simulink model "soc_pmsm_dualcpu_foc_sw_c28xCPU2"  (R2023b)
settings: Solver=FixedStepAuto  StartTime=0.0  StopTime=1  RelTol=1e-3  EnableMultiTasking=on
StartFcn:
  | warning('off', 'Simulink:Engine:ExtModeCannotDownloadParamBecauseNoHostToTarget');
StopFcn:
  | warning('on', 'Simulink:Engine:ExtModeCannotDownloadParamBecauseNoHostToTarget');
undefined symbols (not defined in the file): m, n
libraries: prociodatalib x6, proctasklib x1
settings Model: Creator=13571  LastModifiedBy=13571
settings SolverCC: AlgebraicLoopSolver=TrustRegion  PositivePriorityOrder=on  MaxZcPerStep=1
settings DataIOCC: SaveOutput=off  DSMLogging=off
settings OptimizationCC: DefaultUnderspecifiedDataType=single  EnhancedBackFolding=on  PassReuseOutputArgsAs=Individual arguments  MaxStackSize=1024  OptimizeBlockOrder=speed  DifferentSizesBufferReuse=on  OptimizationCustomize=off  DenormalBehavior=FlushToZero  EfficientTunableParamExpr=on
settings DebuggingCC: InheritedTsInSrcMsg=none  ParameterPrecisionLossMsg=none  ParameterTunabilityLossMsg=error  UnconnectedInputMsg=warning  UnconnectedOutputMsg=warning  UnconnectedLineMsg=warning
settings HardwareCC: ProdBitPerChar=16  ProdBitPerInt=16  ProdBitPerPointer=32  ProdBitPerSizeT=32  ProdBitPerPtrDiffT=32  ProdLargestAtomicInteger=Integer  ProdLargestAtomicFloat=None  ProdWordSize=16  ProdLongLongMode=on  ProdHWDeviceType=Texas Instruments->C2000  HardwareBoardFeatureSet=SoCBlockset
settings ModelReferenceCC: EnableRefExpFcnMdlSchedulingChecks=on  ModelReferenceNumInstancesAllowed=Single
settings SFSimCC: MATLABDynamicMemAlloc=off
settings RTWCC: Description=Embedded Coder  SystemTargetFile=ert.tlc  HardwareBoard=TI Delfino F28379D LaunchPad  TemplateMakefile=ert_default_tmf  Toolchain=Texas Instruments Code Composer Studio (C2000)  DLArmComputeVersion=19.05
settings CodeAppCC: ForceParamTrailComments=on  IgnoreCustomStorageClasses=off  OperatorAnnotations=on  SimulinkDataObjDesc=on  SFDataObjDesc=on  InsertBlockDesc=on
settings ERTTargetCC: CodeReplacementLibrary=TI C28x  ExtModeTransport=4  ExtModeStaticAlloc=on  ExtModeStaticAllocSize=10000  ExtModeMexFile=ext_xcp  ExtModeIntrfLevel=Level2 - Open

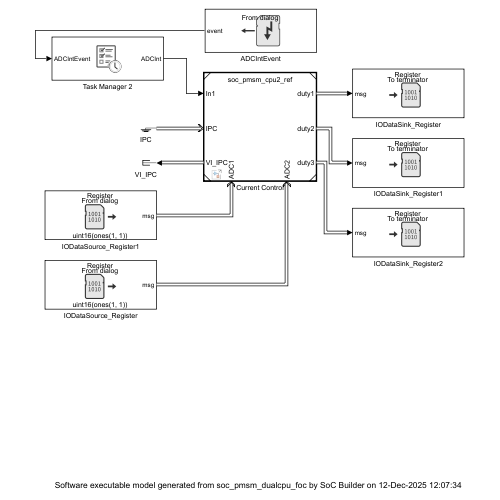
[thumbnail: Simulink's stored preview of the top-level diagram]
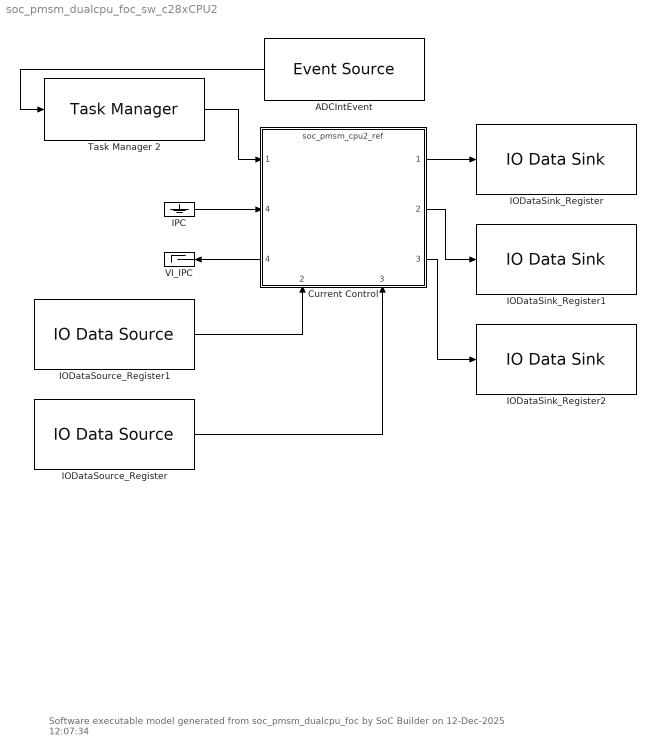
== system soc_pmsm_dualcpu_foc_sw_c28xCPU2 ==
  note: Software executable model generated from soc_pmsm_dualcpu_foc by SoC Builder on 12-Dec-2025 12:07:34
  ADCIntEvent : prociodatalib/Event Source  InputSource=From dialog  ObjectName=[]  SampleTime=-1  Value=1  QueueLength=1  InternalSampleTime=-1
  Current Control : ModelReference  LoadFcn=|  InputPortMessageModes=n,m,m,m  OutputPortMessageModes=m,m,m,m  ModelNameDialog=soc_pmsm_cpu2_ref.slx  SimulationMode=Normal  CachedPortDiscreteRates=[0.2]  ModelReferenceVersion=8.1
      | load_system('soc_pmsm_cpu2_ref');
      | 
      | set_param('soc_pmsm_cpu2_ref', 'Dirty','off');
      settings: PortSchema="{\"entries\":[{\"content\":{\"sides\":[{\"content\":{\"connectorIds\":[\"In1\",\"In4\",\"Out4\"]},\"type\":\"ConnectorPlacement.EquallySpacedRectSide\",\"uuid\":\"9fd2c24c-ae51-46e5-a431-71bc240ed721\"},{\"content\":{\"connectorIds\":[\"Out1\",\"Out2\",\"Out3\"],\"side\":\"RIGHT\"},\"type\":\"ConnectorPlacement.EquallySpacedRectSide\",\"uuid\":\"f0a0e173-5aee-453c-b1bd-b370cde086ab\"},{\"content\":{\"connectorIds\":[],\"side\":\"TOP\"},\"type\":\"ConnectorPlacement.EquallySpacedRectSide\",\"uuid\":\"79c8d290-c938-4b10-a214-67592e778693\"},{\"content\":{\"connectorIds\":[\"In2\",\"In3\"],\"side\":\"BOTTOM\"},\"type\":\"ConnectorPlacement.EquallySpacedRectSide\",\"uuid\":\"f9ab5770-0d25-45e9-9b4a-55a67569c63a\"},{\"content\":{\"connectorIds\":[],\"side\":\"HIDDEN\"},\"type\":\"ConnectorPlacement.EquallySpacedRectSide\",\"uuid\":\"b923878a-78df-441a-99e2-7ad72d4d69ab\"}]},\"type\":\"ConnectorPlacement.EquallySpacedConnector\",\"uuid\":\"a5006b0b-636b-4340-a85c-125b87b251fa\"}],\"packageUris\":[\"http://schema.mathworks.com/mf0/Connector/R2020b\"],\"version\":\"1.0\"}"
  IODataSink_Register : prociodatalib/IO Data Sink  OutputSink=To terminator  DataTypeStr=uint32  Dimensions=1024  DeviceType=Register  EventDataPort=Data  QueueLength=8  SampleTime=-1  EnableDonePort=off
  IODataSink_Register1 : prociodatalib/IO Data Sink  OutputSink=To terminator  DataTypeStr=uint32  Dimensions=1024  DeviceType=Register  EventDataPort=Data  QueueLength=8  SampleTime=-1  EnableDonePort=off
  IODataSink_Register2 : prociodatalib/IO Data Sink  OutputSink=To terminator  DataTypeStr=uint32  Dimensions=1024  DeviceType=Register  EventDataPort=Data  QueueLength=8  SampleTime=-1  EnableDonePort=off
  IODataSource_Register : prociodatalib/IO Data Source  InputSource=From dialog  Value=uint16(ones(1, 1))  ObjectName=[]  DeviceType=Register  ShowEventPort=off  EventDataPort=Data  QueueLength=8  DataTypeStr=uint32  Dimensions=1024  ShowDonePort=off  SampleTime=inf  InternalSampleTime=inf
  IODataSource_Register1 : prociodatalib/IO Data Source  InputSource=From dialog  Value=uint16(ones(1, 1))  ObjectName=[]  DeviceType=Register  ShowEventPort=off  EventDataPort=Data  QueueLength=8  DataTypeStr=uint32  Dimensions=1024  ShowDonePort=off  SampleTime=inf  InternalSampleTime=inf
  IPC : Ground
  Task Manager 2 : proctasklib/Task Manager  AllTaskData="{\"taskName\":\"ADCInt\",\"taskType\":\"Event-driven\",\"taskEvent\":\"ADCIntEvent\",\"taskPeriod\":\"0.1\",\"taskPriority\":\"50\",\"coreSelection\":\"Specified core\",\"coreNum\":\"0\",\"dropOverranTasks\":false,\"playbackRecorded\":false,\"diagnosticsFile\":\"\",\"taskDurationSource\":\"Dialog\",\"taskDuration\":1E-6,\"taskDurationDeviation\":0,\"logExecutionData\":true,\"logDroppedTasks\":false,\"version\":\"2.6\",\"taskDurationData\":{\"percent\":\"100\",\"mean\":\"1e-06\",\"dev\":\"0\",\"min\":\"1e-06\",\"max\":\"1e-06\"},\"taskEventSource\":\"EOC event\",\"taskEventSourceAssignmentType\":\"ManuallyAssigned\",\"taskEventSourceType\":\"Unspecified\",\"taskEventGroup\":\"ADC - Analog to Digital Converter\",\"taskEventInterrupt\":\"ADCB1_INT\",\"taskEventOrder\":1,\"taskDisablePremption\":false,\"taskClearInterruptFlagsAtEndOfEvent\":false}"  EnableTaskSimulation=off  StreamToSDI=on  WriteToFile=off  OverwriteFile=off  SupportEventPorts=on  UseScheduleEditor=off  CustomizationInfo=''
  VI_IPC : Terminator
  wires:
  Current Control/3 -> IODataSink_Register2/1
  Current Control/2 -> IODataSink_Register1/1
  Task Manager 2/1 -> Current Control/1
  IPC/1 -> Current Control/4
  Current Control/4 -> VI_IPC/1
  IODataSource_Register1/1 -> Current Control/2
  IODataSource_Register/1 -> Current Control/3
  ADCIntEvent/1 -> Task Manager 2/1
  Current Control/1 -> IODataSink_Register/1
